simulink model "Base_Map_cs"  (R2019a)
settings: Solver=FixedStepDiscrete  StartTime=0.0  StopTime=15  FixedStep=1/300  RelTol=1e-3
PreLoadFcn:
  | mbxruntime.callbacks.PreLoadFcn(bdroot);
  | check_NUTS_defined
  | model_closed = 0;
  | assignin('base',['model_closed_' bdroot],false);
PostLoadFcn:
  | mbxruntime.callbacks.PostLoadFcn(bdroot);
InitFcn:
  | mbxruntime.callbacks.InitFcn(bdroot);
StartFcn:
  | mbxruntime.callbacks.StartFcn(bdroot);
StopFcn:
  | mbxruntime.callbacks.StopFcn(bdroot);;
  | 
model workspace: external: MAT-File .\Base_Map_S_cs_hws.mat (data not in the file)
undefined symbols (not defined in the file or in its folder): AngularVelocity, Clock_, Data, Data_SL_Info, DiscIntNeverNeededParam, Encoding, Encoding_SL_Info, Header, Height, InitImageOutputDir, LinearAcceleration, mbxruntime, Orientation, Pose, Poses, Poses_SL_Info, Position, Step, tabledata, Twist, Width
libraries: PBCSimulinkLibrary x53, robotlib x26, simulink_extras x19, PreScanSimulinkLibrary x6, dspindex x4, robotcorelib x2, sharedtransform x2, visionconversions x1, visionsinks x1
(part 3 of 8)

== system Base_Map_cs/PointCloudSensor_2 ==
  Sensor : S-Function  FunctionName=sfun_PCS  Parameters=sensorID, dataWidth, dataHeight, numChannels, dataType, timestep  SFunctionDeploymentMode=off  EnableBusSupport=off  mask(PreScan Source Block: Point Cloud Sensor){sensorID=9053, dataWidth=16, dataHeight=900, numChannels=4, dataType=0, timestep=1/20}
      mask prompts: sensorID "Sensor ID"; dataWidth "Data Width"; dataHeight "Data Height"; numChannels "Channel Count"; dataType "Data Type"; timestep "MATLAB timestep:"
      mask help: The Point Cloud Sensor provides XYZ positions relative to the sensor
      mask Help: eval('openHelp(6400)')
      mask Display: image(imread('PointCloudSensorSL.png'))
  PointCloudSensor_2 : Outport  Tag=outport/PointCloudInport  OutDataTypeStr=single  SampleTime=1/20
  wires:
  Sensor/1 -> PointCloudSensor_2/1

== system Base_Map_cs/PointCloudSensor_3 ==
  Sensor : S-Function  FunctionName=sfun_PCS  Parameters=sensorID, dataWidth, dataHeight, numChannels, dataType, timestep  SFunctionDeploymentMode=off  EnableBusSupport=off  mask(PreScan Source Block: Point Cloud Sensor){sensorID=9054, dataWidth=16, dataHeight=900, numChannels=4, dataType=0, timestep=1/20}
      mask prompts: sensorID "Sensor ID"; dataWidth "Data Width"; dataHeight "Data Height"; numChannels "Channel Count"; dataType "Data Type"; timestep "MATLAB timestep:"
      mask help: The Point Cloud Sensor provides XYZ positions relative to the sensor
      mask Help: eval('openHelp(6400)')
      mask Display: image(imread('PointCloudSensorSL.png'))
  PointCloudSensor_3 : Outport  Tag=outport/PointCloudInport  OutDataTypeStr=single  SampleTime=1/20
  wires:
  Sensor/1 -> PointCloudSensor_3/1

== system Base_Map_cs/PointCloudSensor_4 ==
  Sensor : S-Function  FunctionName=sfun_PCS  Parameters=sensorID, dataWidth, dataHeight, numChannels, dataType, timestep  SFunctionDeploymentMode=off  EnableBusSupport=off  mask(PreScan Source Block: Point Cloud Sensor){sensorID=9055, dataWidth=16, dataHeight=900, numChannels=4, dataType=0, timestep=1/20}
      mask prompts: sensorID "Sensor ID"; dataWidth "Data Width"; dataHeight "Data Height"; numChannels "Channel Count"; dataType "Data Type"; timestep "MATLAB timestep:"
      mask help: The Point Cloud Sensor provides XYZ positions relative to the sensor
      mask Help: eval('openHelp(6400)')
      mask Display: image(imread('PointCloudSensorSL.png'))
  PointCloudSensor_4 : Outport  Tag=outport/PointCloudInport  OutDataTypeStr=single  SampleTime=1/20
  wires:
  Sensor/1 -> PointCloudSensor_4/1

== system Base_Map_cs/PreScanTerminator ==
  Terminator : Terminator
  sfun_Terminator : S-Function  FunctionName=sfun_Terminator  Parameters=SampleTime  SFunctionDeploymentMode=off  EnableBusSupport=off  mask(Legacy Function){SFunctionSpec=void prescan_terminator_outputFcn(void ** work1, PRESCAN_TERMINATORDATA y1[1]), SampleTime=TimeStep, ShowSpec=on}
      mask prompts: SampleTime "Sample time (-1 for inherited):"; ShowSpec "Display function specification"
      mask help:
      | This block allows you to call the legacy functions specified by the following Legacy Code Tool definition:
      | def.SFunctionName = 'sfun_Terminator';
      | def.OutputFcnSpec = 'void prescan_terminator_outputFcn(void ** work1, PRESCAN_TERMINATORDATA y1[1])';
      | def.StartFcnSpec = 'void prescan_terminator_startFcn(void ** work1)';
      | def.TerminateFcnSpec = 'void prescan_terminator_terminateFcn(void ** work1)';
      | def.HeaderFiles = {'prescan_terminator_data.h'};
      | def.HostLibFiles = {'sensorinterfaced.lib'};
      | def.IncPaths = {'src', 'C:\prescandev\vislibrary\vis\..\pimp\include\sensors\InterfaceRTW'};
      | def.SrcPaths = {'src'};
      | def.LibPaths = {'C:\\prescandev\\vislibrary_build\lib'};
      | def.SampleTime = 'parameterized';
      | def.Options.language = 'C';
      mask Help: <p>This block was generated automatically by the Legacy Code Tool. For detailed help on this tool, call<a href="matlab:legacy_code('help')"> legacy_code('help')</a>.</p>
      mask Callback ShowSpec:
      | if strcmp(get_param(gcbh, 'ShowSpec'), 'on')
      |   set_param(gcbh, 'MaskDisplay', sprintf('fprintf(''%s'');', get_param(gcbh, 'SFunctionSpec')));
      | else
      |   set_param(gcbh, 'MaskDisplay', sprintf('fprintf(''%s'');', get_param(gcbh, 'FunctionName')));
      | end
      mask Display: fprintf('void prescan_terminator_outputFcn(void ** work1, PRESCAN_TERMINATORDATA y1[1])');
  wires:
  sfun_Terminator/1 -> Terminator/1

== system Base_Map_cs/SELF_BMW_X5_SUV_1 ==
  Sensor : S-Function  FunctionName=sfun_SelfSensor  Parameters=UniqueID, TimeStep  SFunctionDeploymentMode=off  EnableBusSupport=off  mask(PreScan Source Block: SELF){UniqueID=9040, TimeStep=1/300}
      mask prompts: UniqueID "Auto-Assigned: Unique ID"; TimeStep "Auto-Assigned: Upload Period [s]"
      mask help:
      | The SELF port shows (state) information of the actor itself. The outputs are position in the experiment's axis system and the GPS coordinates, and the object's absolute velocity and compass heading.
      |
      | For more information, please click Help.
      mask Help: eval('openHelp(462)')
      mask Display: image(imread('GPS.png'))
  SELF_BMW_X5_SUV_1 : Outport  Tag=outport/SelfPort  OutDataTypeStr=Bus: PRESCAN_SELFSENSORDATA  PortDimensions=1  SampleTime=1/300
  wires:
  Sensor/1 -> SELF_BMW_X5_SUV_1/1

== system Base_Map_cs/SELF_Citroen_C3_Hatchback_1 ==
  Sensor : S-Function  FunctionName=sfun_SelfSensor  Parameters=UniqueID, TimeStep  SFunctionDeploymentMode=off  EnableBusSupport=off  mask(PreScan Source Block: SELF){UniqueID=4877, TimeStep=1/300}
      mask prompts: UniqueID "Auto-Assigned: Unique ID"; TimeStep "Auto-Assigned: Upload Period [s]"
      mask help:
      | The SELF port shows (state) information of the actor itself. The outputs are position in the experiment's axis system and the GPS coordinates, and the object's absolute velocity and compass heading.
      |
      | For more information, please click Help.
      mask Help: eval('openHelp(462)')
      mask Display: image(imread('GPS.png'))
  SELF_Citroen_C3_Hatchback_1 : Outport  Tag=outport/SelfPort  OutDataTypeStr=Bus: PRESCAN_SELFSENSORDATA  PortDimensions=1  SampleTime=1/300
  wires:
  Sensor/1 -> SELF_Citroen_C3_Hatchback_1/1

== system Base_Map_cs/SELF_Ford_Fiesta_Hatchback_1 ==
  Sensor : S-Function  FunctionName=sfun_SelfSensor  Parameters=UniqueID, TimeStep  SFunctionDeploymentMode=off  EnableBusSupport=off  mask(PreScan Source Block: SELF){UniqueID=4876, TimeStep=1/300}
      mask prompts: UniqueID "Auto-Assigned: Unique ID"; TimeStep "Auto-Assigned: Upload Period [s]"
      mask help:
      | The SELF port shows (state) information of the actor itself. The outputs are position in the experiment's axis system and the GPS coordinates, and the object's absolute velocity and compass heading.
      |
      | For more information, please click Help.
      mask Help: eval('openHelp(462)')
      mask Display: image(imread('GPS.png'))
  SELF_Ford_Fiesta_Hatchback_1 : Outport  Tag=outport/SelfPort  OutDataTypeStr=Bus: PRESCAN_SELFSENSORDATA  PortDimensions=1  SampleTime=1/300
  wires:
  Sensor/1 -> SELF_Ford_Fiesta_Hatchback_1/1

== system Base_Map_cs/STATE_BMW_X5_SUV_1_bus ==
  STATE_BMW_X5_SUV_1_bus : Inport  Tag=inport/StatePort  OutDataTypeStr=Bus: PRESCAN_STATEACTUATORDATA  PortDimensions=1  SampleTime=1/300  BusOutputAsStruct=on
  Actuator : S-Function  FunctionName=sfun_StateActuator  Parameters=UniqueID, TimeStep  SFunctionDeploymentMode=off  EnableBusSupport=off  mask(PreScan Sink Block: State){UniqueID=9040, TimeStep=1/300}
      mask prompts: UniqueID "Auto-Assigned: Unique ID"; TimeStep "Auto-Assigned: Upload Period [s]"
      mask help:
      | The Actor State contains a vector signal of size (9x1), containing the following signals:
      |
      | -  Position    	(x,y,z)             	[m]
      | -  Velocity    	(vx,vy,vz)         	[m/s]
      | -  Angles       	(Roll, Pitch, Yaw)	[rad]
      |
      | The Actor state is defined in the global axis system.
      | The state is superponed on the Initial position defined in the GUI.
      |
      | For more information, please click Help.
      mask Help: eval('openHelp(222)')
      mask Display: image(imread('State.png'))
  wires:
  STATE_BMW_X5_SUV_1_bus/1 -> Actuator/1

== system Base_Map_cs/STATE_Citroen_C3_Hatchback_1_bus ==
  STATE_Citroen_C3_Hatchback_1_bus : Inport  Tag=inport/StatePort  OutDataTypeStr=Bus: PRESCAN_STATEACTUATORDATA  PortDimensions=1  SampleTime=1/300  BusOutputAsStruct=on
  Actuator : S-Function  FunctionName=sfun_StateActuator  Parameters=UniqueID, TimeStep  SFunctionDeploymentMode=off  EnableBusSupport=off  mask(PreScan Sink Block: State){UniqueID=4877, TimeStep=1/300}
      mask prompts: UniqueID "Auto-Assigned: Unique ID"; TimeStep "Auto-Assigned: Upload Period [s]"
      mask help:
      | The Actor State contains a vector signal of size (9x1), containing the following signals:
      |
      | -  Position    	(x,y,z)             	[m]
      | -  Velocity    	(vx,vy,vz)         	[m/s]
      | -  Angles       	(Roll, Pitch, Yaw)	[rad]
      |
      | The Actor state is defined in the global axis system.
      | The state is superponed on the Initial position defined in the GUI.
      |
      | For more information, please click Help.
      mask Help: eval('openHelp(222)')
      mask Display: image(imread('State.png'))
  wires:
  STATE_Citroen_C3_Hatchback_1_bus/1 -> Actuator/1

== system Base_Map_cs/STATE_Ford_Fiesta_Hatchback_1_bus ==
  STATE_Ford_Fiesta_Hatchback_1_bus : Inport  Tag=inport/StatePort  OutDataTypeStr=Bus: PRESCAN_STATEACTUATORDATA  PortDimensions=1  SampleTime=1/300  BusOutputAsStruct=on
  Actuator : S-Function  FunctionName=sfun_StateActuator  Parameters=UniqueID, TimeStep  SFunctionDeploymentMode=off  EnableBusSupport=off  mask(PreScan Sink Block: State){UniqueID=4876, TimeStep=1/300}
      mask prompts: UniqueID "Auto-Assigned: Unique ID"; TimeStep "Auto-Assigned: Upload Period [s]"
      mask help:
      | The Actor State contains a vector signal of size (9x1), containing the following signals:
      |
      | -  Position    	(x,y,z)             	[m]
      | -  Velocity    	(vx,vy,vz)         	[m/s]
      | -  Angles       	(Roll, Pitch, Yaw)	[rad]
      |
      | The Actor state is defined in the global axis system.
      | The state is superponed on the Initial position defined in the GUI.
      |
      | For more information, please click Help.
      mask Help: eval('openHelp(222)')
      mask Display: image(imread('State.png'))
  wires:
  STATE_Ford_Fiesta_Hatchback_1_bus/1 -> Actuator/1

== system Base_Map_cs/Synchronizer ==
  Bus Selector1 : BusSelector  OutputSignals=FederateStopped
  Stop Simulation : Stop
  sfun_Synchronizer : S-Function  FunctionName=sfun_Synchronizer  Parameters=SampleTime  SFunctionDeploymentMode=off  EnableBusSupport=off  mask(Legacy Function){SFunctionSpec=void prescan_synchronizer_outputFcn(void ** work1, PRESCAN_SYNCHRONIZEDATA y1[1]), SampleTime=TimeStep, ShowSpec=on}
      mask prompts: SampleTime "Sample time (-1 for inherited):"; ShowSpec "Display function specification"
      mask help:
      | This block allows you to call the legacy functions specified by the following Legacy Code Tool definition:
      | def.SFunctionName = 'sfun_Synchronizer';
      | def.OutputFcnSpec = 'void prescan_synchronizer_outputFcn(void ** work1, PRESCAN_SYNCHRONIZEDATA y1[1])';
      | def.StartFcnSpec = 'void prescan_synchronizer_startFcn(void ** work1)';
      | def.TerminateFcnSpec = 'void prescan_synchronizer_terminateFcn(void ** work1)';
      | def.HeaderFiles = {'prescan_synchronizer_data.h'};
      | def.HostLibFiles = {'sensorinterfaced.lib'};
      | def.IncPaths = {'src', 'C:\prescandev\vislibrary\vis\..\pimp\include\sensors\InterfaceRTW'};
      | def.SrcPaths = {'src'};
      | def.LibPaths = {'C:\\prescandev\\vislibrary_build\lib'};
      | def.SampleTime = 'parameterized';
      | def.Options.language = 'C';
      mask Help: <p>This block was generated automatically by the Legacy Code Tool. For detailed help on this tool, call<a href="matlab:legacy_code('help')"> legacy_code('help')</a>.</p>
      mask Callback ShowSpec:
      | if strcmp(get_param(gcbh, 'ShowSpec'), 'on')
      |   set_param(gcbh, 'MaskDisplay', sprintf('fprintf(''%s'');', get_param(gcbh, 'SFunctionSpec')));
      | else
      |   set_param(gcbh, 'MaskDisplay', sprintf('fprintf(''%s'');', get_param(gcbh, 'FunctionName')));
      | end
      mask Display: fprintf('void prescan_synchronizer_outputFcn(void ** work1, PRESCAN_SYNCHRONIZEDATA y1[1])');
  wires:
  Bus Selector1/1 -> Stop Simulation/1  "<FederateStopped>"
  sfun_Synchronizer/1 -> Bus Selector1/1

== system Base_Map_cs/TrafficLightRoadSideNL_1 ==
  note: Light SPD Resources
      |
      |  0: CIE_A_standard_incandescent_illuminant.txt
      |  1: CIE_A_standard_incandescent_illuminant.txt_x_R255_G191_B000.txt
      |  2: CIE_A_standard_incandescent_illuminant.txt_x_R583_G047_B000.txt
      |  3: CIE_F12_standard_fluorescent_illuminant.txt
      |  4: Illuminant_D65.txt
      |  5: Light_SPD_H1_12_8V_Filament.txt
      |  6: Light_SPD_H1_13_2V_Filament.txt
      |  7: Light_SPD_H11_12V_Filament.txt
      |  8: Light_SPD_H7_12_8V_Filament.txt
      |  9: Light_SPD_H7_13_2V_Filament.txt
      | 10: Light_SPD_H8_13_2V_Filament.txt
      | 11: Light_SPD_Halogen.txt
      | 12: Light_SPD_High_Power_LED.txt
      | 13: Light_SPD_HPS_High_Pressure_Sodium.txt
      | 14: Light_SPD_incandescent_traffic_signal_amber.txt
      | 15: Light_SPD_incandescent_traffic_signal_green.txt
      | 16: Light_SPD_incandescent_traffic_signal_red.txt
      | 17: Light_SPD_LED_D1S_HID.txt
      | 18: Light_SPD_LED_traffic_signal_amber.txt
      | 19: Light_SPD_LED_traffic_signal_green.txt
      | 20: Light_SPD_LED_traffic_signal_red.txt
      | 21: Light_SPD_LPS_Low_Pressure_Sodium.txt
      | 22: Light_SPD_Mercury.txt
      | 23: Light_SPD_Reddish_Neon_Sign.txt
      | 24: Noma_Twister_Blue_13W_120V.txt
      | 25: Philips_Blue_Golite_P1_Apollo_1750Lux.txt
      | 26: SPD_flat_1.0.txt
  note: Light SPD Resources
  Ground_1 : Ground
  Ground_2 : Ground
  Ground_3 : Ground
  TrafficLightRoadSideNL_1_Casing.LightGreen_Control_Mux : Subsystem  Tag=mux/plugin/LightSignals
  TrafficLightRoadSideNL_1_Casing.LightGreen_Power : Constant  Tag=TrafficLightRoadSideNL_1_Casing.LightGreen_Power  Value=0
  TrafficLightRoadSideNL_1_Casing.LightGreen_SPDIndex : Constant  Tag=TrafficLightRoadSideNL_1_Casing.LightGreen_SPDIndex  Value=15
  TrafficLightRoadSideNL_1_Casing.LightOrange_Control_Mux : Subsystem  Tag=mux/plugin/LightSignals
  TrafficLightRoadSideNL_1_Casing.LightOrange_Power : Constant  Tag=TrafficLightRoadSideNL_1_Casing.LightOrange_Power  Value=0
  TrafficLightRoadSideNL_1_Casing.LightOrange_SPDIndex : Constant  Tag=TrafficLightRoadSideNL_1_Casing.LightOrange_SPDIndex  Value=14
  TrafficLightRoadSideNL_1_Casing.LightRed_Control_Mux : Subsystem  Tag=mux/plugin/LightSignals
  TrafficLightRoadSideNL_1_Casing.LightRed_Power : Constant  Tag=TrafficLightRoadSideNL_1_Casing.LightRed_Power  Value=0
  TrafficLightRoadSideNL_1_Casing.LightRed_SPDIndex : Constant  Tag=TrafficLightRoadSideNL_1_Casing.LightRed_SPDIndex  Value=16
  VISUCasingLights_Mux : Subsystem  Tag=mux/VisuCasingLights  mask(PreScan User Interface: VisuTrafficLight){}
      mask help:
      | The VisuTrafficLight block provides a way to animate traffic lights: switch on and off individual lights.
      |
      | For more information, please click Help.
      mask Help: eval('openHelp(731)')
  VISUCasingLights_TrafficLightRoadSideNL_1 : Outport  Tag=outport/VisuCasingLights  SampleTime=1/300
  TrafficLightRoadSideNL_1_Casing.LightRed_Control : Outport  Tag=outport/plugin/sfun_PBCLight  Port=2  OutDataTypeStr=Bus: PRESCAN_PBCLIGHT_DATA  PortDimensions=1  SampleTime=0.05
  TrafficLightRoadSideNL_1_Casing.LightOrange_Control : Outport  Tag=outport/plugin/sfun_PBCLight  Port=3  OutDataTypeStr=Bus: PRESCAN_PBCLIGHT_DATA  PortDimensions=1  SampleTime=0.05
  TrafficLightRoadSideNL_1_Casing.LightGreen_Control : Outport  Tag=outport/plugin/sfun_PBCLight  Port=4  OutDataTypeStr=Bus: PRESCAN_PBCLIGHT_DATA  PortDimensions=1  SampleTime=0.05
  wires:
  VISUCasingLights_Mux/1(VISUCasingLights_TrafficLightRoadSideNL_1) -> VISUCasingLights_TrafficLightRoadSideNL_1/1
  TrafficLightRoadSideNL_1_Casing.LightRed_Control_Mux/1(Bus) -> TrafficLightRoadSideNL_1_Casing.LightRed_Control/1
  TrafficLightRoadSideNL_1_Casing.LightRed_SPDIndex/1 -> TrafficLightRoadSideNL_1_Casing.LightRed_Control_Mux/1(SPDIndex [-])
  TrafficLightRoadSideNL_1_Casing.LightRed_Power/1 -> TrafficLightRoadSideNL_1_Casing.LightRed_Control_Mux/2(Power [W])
  TrafficLightRoadSideNL_1_Casing.LightOrange_Control_Mux/1(Bus) -> TrafficLightRoadSideNL_1_Casing.LightOrange_Control/1
  TrafficLightRoadSideNL_1_Casing.LightOrange_SPDIndex/1 -> TrafficLightRoadSideNL_1_Casing.LightOrange_Control_Mux/1(SPDIndex [-])
  TrafficLightRoadSideNL_1_Casing.LightOrange_Power/1 -> TrafficLightRoadSideNL_1_Casing.LightOrange_Control_Mux/2(Power [W])
  TrafficLightRoadSideNL_1_Casing.LightGreen_Control_Mux/1(Bus) -> TrafficLightRoadSideNL_1_Casing.LightGreen_Control/1
  TrafficLightRoadSideNL_1_Casing.LightGreen_SPDIndex/1 -> TrafficLightRoadSideNL_1_Casing.LightGreen_Control_Mux/1(SPDIndex [-])
  TrafficLightRoadSideNL_1_Casing.LightGreen_Power/1 -> TrafficLightRoadSideNL_1_Casing.LightGreen_Control_Mux/2(Power [W])
  Ground_1/1 -> VISUCasingLights_Mux/1(Green [-])
  Ground_2/1 -> VISUCasingLights_Mux/2(Orange [-])
  Ground_3/1 -> VISUCasingLights_Mux/3(Red [-])

== system Base_Map_cs/TrafficLightRoadSideNL_1_Casing.LightGreen_Control ==
  TrafficLightRoadSideNL_1_Casing.LightGreen_Control : Inport  Tag=inport/plugin/sfun_PBCLight  OutDataTypeStr=Bus: PRESCAN_PBCLIGHT_DATA  PortDimensions=1  SampleTime=0.05  BusOutputAsStruct=on
  Actuator : S-Function  LoadFcn=addpath 'C:/Program Files/Simcenter Prescan/Prescan_2019.1/Plugins/PBCameraPlugin/matlab';addpath 'C:/Program Files/Simcenter Prescan/Prescan_2019.1/Plugins/PBCameraPlugin/bin';load('PreScanPBCLightData.mat');  FunctionName=sfun_PBCLight  Parameters=lightID, timestepMask  SFunctionDeploymentMode=off  EnableBusSupport=off  mask(Physics Based Camera plugin block){lightID=2, timestepMask=0.05}
      mask prompts: lightID "Light ID:"; timestepMask "MATLAB timestep:"
      mask help: Light Control I/O
      mask Help: eval('openHelp(6500)')
      mask Display: image(imread('ico_PBCControl.png'))
  wires:
  TrafficLightRoadSideNL_1_Casing.LightGreen_Control/1 -> Actuator/1

== system Base_Map_cs/TrafficLightRoadSideNL_1_Casing.LightOrange_Control ==
  TrafficLightRoadSideNL_1_Casing.LightOrange_Control : Inport  Tag=inport/plugin/sfun_PBCLight  OutDataTypeStr=Bus: PRESCAN_PBCLIGHT_DATA  PortDimensions=1  SampleTime=0.05  BusOutputAsStruct=on
  Actuator : S-Function  LoadFcn=addpath 'C:/Program Files/Simcenter Prescan/Prescan_2019.1/Plugins/PBCameraPlugin/matlab';addpath 'C:/Program Files/Simcenter Prescan/Prescan_2019.1/Plugins/PBCameraPlugin/bin';load('PreScanPBCLightData.mat');  FunctionName=sfun_PBCLight  Parameters=lightID, timestepMask  SFunctionDeploymentMode=off  EnableBusSupport=off  mask(Physics Based Camera plugin block){lightID=1, timestepMask=0.05}
      mask prompts: lightID "Light ID:"; timestepMask "MATLAB timestep:"
      mask help: Light Control I/O
      mask Help: eval('openHelp(6500)')
      mask Display: image(imread('ico_PBCControl.png'))
  wires:
  TrafficLightRoadSideNL_1_Casing.LightOrange_Control/1 -> Actuator/1

== system Base_Map_cs/TrafficLightRoadSideNL_1_Casing.LightRed_Control ==
  TrafficLightRoadSideNL_1_Casing.LightRed_Control : Inport  Tag=inport/plugin/sfun_PBCLight  OutDataTypeStr=Bus: PRESCAN_PBCLIGHT_DATA  PortDimensions=1  SampleTime=0.05  BusOutputAsStruct=on
  Actuator : S-Function  LoadFcn=addpath 'C:/Program Files/Simcenter Prescan/Prescan_2019.1/Plugins/PBCameraPlugin/matlab';addpath 'C:/Program Files/Simcenter Prescan/Prescan_2019.1/Plugins/PBCameraPlugin/bin';load('PreScanPBCLightData.mat');  FunctionName=sfun_PBCLight  Parameters=lightID, timestepMask  SFunctionDeploymentMode=off  EnableBusSupport=off  mask(Physics Based Camera plugin block){lightID=0, timestepMask=0.05}
      mask prompts: lightID "Light ID:"; timestepMask "MATLAB timestep:"
      mask help: Light Control I/O
      mask Help: eval('openHelp(6500)')
      mask Display: image(imread('ico_PBCControl.png'))
  wires:
  TrafficLightRoadSideNL_1_Casing.LightRed_Control/1 -> Actuator/1

== system Base_Map_cs/TrafficLightRoadSideNL_2 ==
  note: Light SPD Resources
      |
      |  0: CIE_A_standard_incandescent_illuminant.txt
      |  1: CIE_A_standard_incandescent_illuminant.txt_x_R255_G191_B000.txt
      |  2: CIE_A_standard_incandescent_illuminant.txt_x_R583_G047_B000.txt
      |  3: CIE_F12_standard_fluorescent_illuminant.txt
      |  4: Illuminant_D65.txt
      |  5: Light_SPD_H1_12_8V_Filament.txt
      |  6: Light_SPD_H1_13_2V_Filament.txt
      |  7: Light_SPD_H11_12V_Filament.txt
      |  8: Light_SPD_H7_12_8V_Filament.txt
      |  9: Light_SPD_H7_13_2V_Filament.txt
      | 10: Light_SPD_H8_13_2V_Filament.txt
      | 11: Light_SPD_Halogen.txt
      | 12: Light_SPD_High_Power_LED.txt
      | 13: Light_SPD_HPS_High_Pressure_Sodium.txt
      | 14: Light_SPD_incandescent_traffic_signal_amber.txt
      | 15: Light_SPD_incandescent_traffic_signal_green.txt
      | 16: Light_SPD_incandescent_traffic_signal_red.txt
      | 17: Light_SPD_LED_D1S_HID.txt
      | 18: Light_SPD_LED_traffic_signal_amber.txt
      | 19: Light_SPD_LED_traffic_signal_green.txt
      | 20: Light_SPD_LED_traffic_signal_red.txt
      | 21: Light_SPD_LPS_Low_Pressure_Sodium.txt
      | 22: Light_SPD_Mercury.txt
      | 23: Light_SPD_Reddish_Neon_Sign.txt
      | 24: Noma_Twister_Blue_13W_120V.txt
      | 25: Philips_Blue_Golite_P1_Apollo_1750Lux.txt
      | 26: SPD_flat_1.0.txt
  note: Light SPD Resources
  Ground_1 : Ground
  Ground_2 : Ground
  Ground_3 : Ground
  TrafficLightRoadSideNL_2_Casing.LightGreen_Control_Mux : Subsystem  Tag=mux/plugin/LightSignals
  TrafficLightRoadSideNL_2_Casing.LightGreen_Power : Constant  Tag=TrafficLightRoadSideNL_2_Casing.LightGreen_Power  Value=0
  TrafficLightRoadSideNL_2_Casing.LightGreen_SPDIndex : Constant  Tag=TrafficLightRoadSideNL_2_Casing.LightGreen_SPDIndex  Value=15
  TrafficLightRoadSideNL_2_Casing.LightOrange_Control_Mux : Subsystem  Tag=mux/plugin/LightSignals
  TrafficLightRoadSideNL_2_Casing.LightOrange_Power : Constant  Tag=TrafficLightRoadSideNL_2_Casing.LightOrange_Power  Value=0
  TrafficLightRoadSideNL_2_Casing.LightOrange_SPDIndex : Constant  Tag=TrafficLightRoadSideNL_2_Casing.LightOrange_SPDIndex  Value=14
  TrafficLightRoadSideNL_2_Casing.LightRed_Control_Mux : Subsystem  Tag=mux/plugin/LightSignals
  TrafficLightRoadSideNL_2_Casing.LightRed_Power : Constant  Tag=TrafficLightRoadSideNL_2_Casing.LightRed_Power  Value=0
  TrafficLightRoadSideNL_2_Casing.LightRed_SPDIndex : Constant  Tag=TrafficLightRoadSideNL_2_Casing.LightRed_SPDIndex  Value=16
  VISUCasingLights_Mux : Subsystem  Tag=mux/VisuCasingLights  mask(PreScan User Interface: VisuTrafficLight){}
      mask help:
      | The VisuTrafficLight block provides a way to animate traffic lights: switch on and off individual lights.
      |
      | For more information, please click Help.
      mask Help: eval('openHelp(731)')
  VISUCasingLights_TrafficLightRoadSideNL_2 : Outport  Tag=outport/VisuCasingLights  SampleTime=1/300
  TrafficLightRoadSideNL_2_Casing.LightRed_Control : Outport  Tag=outport/plugin/sfun_PBCLight  Port=2  OutDataTypeStr=Bus: PRESCAN_PBCLIGHT_DATA  PortDimensions=1  SampleTime=0.05
  TrafficLightRoadSideNL_2_Casing.LightOrange_Control : Outport  Tag=outport/plugin/sfun_PBCLight  Port=3  OutDataTypeStr=Bus: PRESCAN_PBCLIGHT_DATA  PortDimensions=1  SampleTime=0.05
  TrafficLightRoadSideNL_2_Casing.LightGreen_Control : Outport  Tag=outport/plugin/sfun_PBCLight  Port=4  OutDataTypeStr=Bus: PRESCAN_PBCLIGHT_DATA  PortDimensions=1  SampleTime=0.05
  wires:
  VISUCasingLights_Mux/1(VISUCasingLights_TrafficLightRoadSideNL_2) -> VISUCasingLights_TrafficLightRoadSideNL_2/1
  TrafficLightRoadSideNL_2_Casing.LightRed_Control_Mux/1(Bus) -> TrafficLightRoadSideNL_2_Casing.LightRed_Control/1
  TrafficLightRoadSideNL_2_Casing.LightRed_SPDIndex/1 -> TrafficLightRoadSideNL_2_Casing.LightRed_Control_Mux/1(SPDIndex [-])
  TrafficLightRoadSideNL_2_Casing.LightRed_Power/1 -> TrafficLightRoadSideNL_2_Casing.LightRed_Control_Mux/2(Power [W])
  TrafficLightRoadSideNL_2_Casing.LightOrange_Control_Mux/1(Bus) -> TrafficLightRoadSideNL_2_Casing.LightOrange_Control/1
  TrafficLightRoadSideNL_2_Casing.LightOrange_SPDIndex/1 -> TrafficLightRoadSideNL_2_Casing.LightOrange_Control_Mux/1(SPDIndex [-])
  TrafficLightRoadSideNL_2_Casing.LightOrange_Power/1 -> TrafficLightRoadSideNL_2_Casing.LightOrange_Control_Mux/2(Power [W])
  TrafficLightRoadSideNL_2_Casing.LightGreen_Control_Mux/1(Bus) -> TrafficLightRoadSideNL_2_Casing.LightGreen_Control/1
  TrafficLightRoadSideNL_2_Casing.LightGreen_SPDIndex/1 -> TrafficLightRoadSideNL_2_Casing.LightGreen_Control_Mux/1(SPDIndex [-])
  TrafficLightRoadSideNL_2_Casing.LightGreen_Power/1 -> TrafficLightRoadSideNL_2_Casing.LightGreen_Control_Mux/2(Power [W])
  Ground_1/1 -> VISUCasingLights_Mux/1(Green [-])
  Ground_2/1 -> VISUCasingLights_Mux/2(Orange [-])
  Ground_3/1 -> VISUCasingLights_Mux/3(Red [-])

== system Base_Map_cs/TrafficLightRoadSideNL_2_Casing.LightGreen_Control ==
  TrafficLightRoadSideNL_2_Casing.LightGreen_Control : Inport  Tag=inport/plugin/sfun_PBCLight  OutDataTypeStr=Bus: PRESCAN_PBCLIGHT_DATA  PortDimensions=1  SampleTime=0.05  BusOutputAsStruct=on
  Actuator : S-Function  LoadFcn=addpath 'C:/Program Files/Simcenter Prescan/Prescan_2019.1/Plugins/PBCameraPlugin/matlab';addpath 'C:/Program Files/Simcenter Prescan/Prescan_2019.1/Plugins/PBCameraPlugin/bin';load('PreScanPBCLightData.mat');  FunctionName=sfun_PBCLight  Parameters=lightID, timestepMask  SFunctionDeploymentMode=off  EnableBusSupport=off  mask(Physics Based Camera plugin block){lightID=5, timestepMask=0.05}
      mask prompts: lightID "Light ID:"; timestepMask "MATLAB timestep:"
      mask help: Light Control I/O
      mask Help: eval('openHelp(6500)')
      mask Display: image(imread('ico_PBCControl.png'))
  wires:
  TrafficLightRoadSideNL_2_Casing.LightGreen_Control/1 -> Actuator/1

== system Base_Map_cs/TrafficLightRoadSideNL_2_Casing.LightOrange_Control ==
  TrafficLightRoadSideNL_2_Casing.LightOrange_Control : Inport  Tag=inport/plugin/sfun_PBCLight  OutDataTypeStr=Bus: PRESCAN_PBCLIGHT_DATA  PortDimensions=1  SampleTime=0.05  BusOutputAsStruct=on
  Actuator : S-Function  LoadFcn=addpath 'C:/Program Files/Simcenter Prescan/Prescan_2019.1/Plugins/PBCameraPlugin/matlab';addpath 'C:/Program Files/Simcenter Prescan/Prescan_2019.1/Plugins/PBCameraPlugin/bin';load('PreScanPBCLightData.mat');  FunctionName=sfun_PBCLight  Parameters=lightID, timestepMask  SFunctionDeploymentMode=off  EnableBusSupport=off  mask(Physics Based Camera plugin block){lightID=4, timestepMask=0.05}
      mask prompts: lightID "Light ID:"; timestepMask "MATLAB timestep:"
      mask help: Light Control I/O
      mask Help: eval('openHelp(6500)')
      mask Display: image(imread('ico_PBCControl.png'))
  wires:
  TrafficLightRoadSideNL_2_Casing.LightOrange_Control/1 -> Actuator/1

== system Base_Map_cs/TrafficLightRoadSideNL_2_Casing.LightRed_Control ==
  TrafficLightRoadSideNL_2_Casing.LightRed_Control : Inport  Tag=inport/plugin/sfun_PBCLight  OutDataTypeStr=Bus: PRESCAN_PBCLIGHT_DATA  PortDimensions=1  SampleTime=0.05  BusOutputAsStruct=on
  Actuator : S-Function  LoadFcn=addpath 'C:/Program Files/Simcenter Prescan/Prescan_2019.1/Plugins/PBCameraPlugin/matlab';addpath 'C:/Program Files/Simcenter Prescan/Prescan_2019.1/Plugins/PBCameraPlugin/bin';load('PreScanPBCLightData.mat');  FunctionName=sfun_PBCLight  Parameters=lightID, timestepMask  SFunctionDeploymentMode=off  EnableBusSupport=off  mask(Physics Based Camera plugin block){lightID=3, timestepMask=0.05}
      mask prompts: lightID "Light ID:"; timestepMask "MATLAB timestep:"
      mask help: Light Control I/O
      mask Help: eval('openHelp(6500)')
      mask Display: image(imread('ico_PBCControl.png'))
  wires:
  TrafficLightRoadSideNL_2_Casing.LightRed_Control/1 -> Actuator/1

== system Base_Map_cs/TrafficLightRoadSideNL_3 ==
  note: Light SPD Resources
      |
      |  0: CIE_A_standard_incandescent_illuminant.txt
      |  1: CIE_A_standard_incandescent_illuminant.txt_x_R255_G191_B000.txt
      |  2: CIE_A_standard_incandescent_illuminant.txt_x_R583_G047_B000.txt
      |  3: CIE_F12_standard_fluorescent_illuminant.txt
      |  4: Illuminant_D65.txt
      |  5: Light_SPD_H1_12_8V_Filament.txt
      |  6: Light_SPD_H1_13_2V_Filament.txt
      |  7: Light_SPD_H11_12V_Filament.txt
      |  8: Light_SPD_H7_12_8V_Filament.txt
      |  9: Light_SPD_H7_13_2V_Filament.txt
      | 10: Light_SPD_H8_13_2V_Filament.txt
      | 11: Light_SPD_Halogen.txt
      | 12: Light_SPD_High_Power_LED.txt
      | 13: Light_SPD_HPS_High_Pressure_Sodium.txt
      | 14: Light_SPD_incandescent_traffic_signal_amber.txt
      | 15: Light_SPD_incandescent_traffic_signal_green.txt
      | 16: Light_SPD_incandescent_traffic_signal_red.txt
      | 17: Light_SPD_LED_D1S_HID.txt
      | 18: Light_SPD_LED_traffic_signal_amber.txt
      | 19: Light_SPD_LED_traffic_signal_green.txt
      | 20: Light_SPD_LED_traffic_signal_red.txt
      | 21: Light_SPD_LPS_Low_Pressure_Sodium.txt
      | 22: Light_SPD_Mercury.txt
      | 23: Light_SPD_Reddish_Neon_Sign.txt
      | 24: Noma_Twister_Blue_13W_120V.txt
      | 25: Philips_Blue_Golite_P1_Apollo_1750Lux.txt
      | 26: SPD_flat_1.0.txt
  note: Light SPD Resources
  Ground_1 : Ground
  Ground_2 : Ground
  Ground_3 : Ground
  TrafficLightRoadSideNL_3_Casing.LightGreen_Control_Mux : Subsystem  Tag=mux/plugin/LightSignals
  TrafficLightRoadSideNL_3_Casing.LightGreen_Power : Constant  Tag=TrafficLightRoadSideNL_3_Casing.LightGreen_Power  Value=0
  TrafficLightRoadSideNL_3_Casing.LightGreen_SPDIndex : Constant  Tag=TrafficLightRoadSideNL_3_Casing.LightGreen_SPDIndex  Value=15
  TrafficLightRoadSideNL_3_Casing.LightOrange_Control_Mux : Subsystem  Tag=mux/plugin/LightSignals
  TrafficLightRoadSideNL_3_Casing.LightOrange_Power : Constant  Tag=TrafficLightRoadSideNL_3_Casing.LightOrange_Power  Value=0
  TrafficLightRoadSideNL_3_Casing.LightOrange_SPDIndex : Constant  Tag=TrafficLightRoadSideNL_3_Casing.LightOrange_SPDIndex  Value=14
  TrafficLightRoadSideNL_3_Casing.LightRed_Control_Mux : Subsystem  Tag=mux/plugin/LightSignals
  TrafficLightRoadSideNL_3_Casing.LightRed_Power : Constant  Tag=TrafficLightRoadSideNL_3_Casing.LightRed_Power  Value=0
  TrafficLightRoadSideNL_3_Casing.LightRed_SPDIndex : Constant  Tag=TrafficLightRoadSideNL_3_Casing.LightRed_SPDIndex  Value=16
  VISUCasingLights_Mux : Subsystem  Tag=mux/VisuCasingLights  mask(PreScan User Interface: VisuTrafficLight){}
      mask help:
      | The VisuTrafficLight block provides a way to animate traffic lights: switch on and off individual lights.
      |
      | For more information, please click Help.
      mask Help: eval('openHelp(731)')
  VISUCasingLights_TrafficLightRoadSideNL_3 : Outport  Tag=outport/VisuCasingLights  SampleTime=1/300
  TrafficLightRoadSideNL_3_Casing.LightRed_Control : Outport  Tag=outport/plugin/sfun_PBCLight  Port=2  OutDataTypeStr=Bus: PRESCAN_PBCLIGHT_DATA  PortDimensions=1  SampleTime=0.05
  TrafficLightRoadSideNL_3_Casing.LightOrange_Control : Outport  Tag=outport/plugin/sfun_PBCLight  Port=3  OutDataTypeStr=Bus: PRESCAN_PBCLIGHT_DATA  PortDimensions=1  SampleTime=0.05
  TrafficLightRoadSideNL_3_Casing.LightGreen_Control : Outport  Tag=outport/plugin/sfun_PBCLight  Port=4  OutDataTypeStr=Bus: PRESCAN_PBCLIGHT_DATA  PortDimensions=1  SampleTime=0.05
  wires:
  VISUCasingLights_Mux/1(VISUCasingLights_TrafficLightRoadSideNL_3) -> VISUCasingLights_TrafficLightRoadSideNL_3/1
  TrafficLightRoadSideNL_3_Casing.LightRed_Control_Mux/1(Bus) -> TrafficLightRoadSideNL_3_Casing.LightRed_Control/1
  TrafficLightRoadSideNL_3_Casing.LightRed_SPDIndex/1 -> TrafficLightRoadSideNL_3_Casing.LightRed_Control_Mux/1(SPDIndex [-])
  TrafficLightRoadSideNL_3_Casing.LightRed_Power/1 -> TrafficLightRoadSideNL_3_Casing.LightRed_Control_Mux/2(Power [W])
  TrafficLightRoadSideNL_3_Casing.LightOrange_Control_Mux/1(Bus) -> TrafficLightRoadSideNL_3_Casing.LightOrange_Control/1
  TrafficLightRoadSideNL_3_Casing.LightOrange_SPDIndex/1 -> TrafficLightRoadSideNL_3_Casing.LightOrange_Control_Mux/1(SPDIndex [-])
  TrafficLightRoadSideNL_3_Casing.LightOrange_Power/1 -> TrafficLightRoadSideNL_3_Casing.LightOrange_Control_Mux/2(Power [W])
  TrafficLightRoadSideNL_3_Casing.LightGreen_Control_Mux/1(Bus) -> TrafficLightRoadSideNL_3_Casing.LightGreen_Control/1
  TrafficLightRoadSideNL_3_Casing.LightGreen_SPDIndex/1 -> TrafficLightRoadSideNL_3_Casing.LightGreen_Control_Mux/1(SPDIndex [-])
  TrafficLightRoadSideNL_3_Casing.LightGreen_Power/1 -> TrafficLightRoadSideNL_3_Casing.LightGreen_Control_Mux/2(Power [W])
  Ground_1/1 -> VISUCasingLights_Mux/1(Green [-])
  Ground_2/1 -> VISUCasingLights_Mux/2(Orange [-])
  Ground_3/1 -> VISUCasingLights_Mux/3(Red [-])

== system Base_Map_cs/TrafficLightRoadSideNL_3_Casing.LightGreen_Control ==
  TrafficLightRoadSideNL_3_Casing.LightGreen_Control : Inport  Tag=inport/plugin/sfun_PBCLight  OutDataTypeStr=Bus: PRESCAN_PBCLIGHT_DATA  PortDimensions=1  SampleTime=0.05  BusOutputAsStruct=on
  Actuator : S-Function  LoadFcn=addpath 'C:/Program Files/Simcenter Prescan/Prescan_2019.1/Plugins/PBCameraPlugin/matlab';addpath 'C:/Program Files/Simcenter Prescan/Prescan_2019.1/Plugins/PBCameraPlugin/bin';load('PreScanPBCLightData.mat');  FunctionName=sfun_PBCLight  Parameters=lightID, timestepMask  SFunctionDeploymentMode=off  EnableBusSupport=off  mask(Physics Based Camera plugin block){lightID=8, timestepMask=0.05}
      mask prompts: lightID "Light ID:"; timestepMask "MATLAB timestep:"
      mask help: Light Control I/O
      mask Help: eval('openHelp(6500)')
      mask Display: image(imread('ico_PBCControl.png'))
  wires:
  TrafficLightRoadSideNL_3_Casing.LightGreen_Control/1 -> Actuator/1

== system Base_Map_cs/TrafficLightRoadSideNL_3_Casing.LightOrange_Control ==
  TrafficLightRoadSideNL_3_Casing.LightOrange_Control : Inport  Tag=inport/plugin/sfun_PBCLight  OutDataTypeStr=Bus: PRESCAN_PBCLIGHT_DATA  PortDimensions=1  SampleTime=0.05  BusOutputAsStruct=on
  Actuator : S-Function  LoadFcn=addpath 'C:/Program Files/Simcenter Prescan/Prescan_2019.1/Plugins/PBCameraPlugin/matlab';addpath 'C:/Program Files/Simcenter Prescan/Prescan_2019.1/Plugins/PBCameraPlugin/bin';load('PreScanPBCLightData.mat');  FunctionName=sfun_PBCLight  Parameters=lightID, timestepMask  SFunctionDeploymentMode=off  EnableBusSupport=off  mask(Physics Based Camera plugin block){lightID=7, timestepMask=0.05}
      mask prompts: lightID "Light ID:"; timestepMask "MATLAB timestep:"
      mask help: Light Control I/O
      mask Help: eval('openHelp(6500)')
      mask Display: image(imread('ico_PBCControl.png'))
  wires:
  TrafficLightRoadSideNL_3_Casing.LightOrange_Control/1 -> Actuator/1

== system Base_Map_cs/TrafficLightRoadSideNL_3_Casing.LightRed_Control ==
  TrafficLightRoadSideNL_3_Casing.LightRed_Control : Inport  Tag=inport/plugin/sfun_PBCLight  OutDataTypeStr=Bus: PRESCAN_PBCLIGHT_DATA  PortDimensions=1  SampleTime=0.05  BusOutputAsStruct=on
  Actuator : S-Function  LoadFcn=addpath 'C:/Program Files/Simcenter Prescan/Prescan_2019.1/Plugins/PBCameraPlugin/matlab';addpath 'C:/Program Files/Simcenter Prescan/Prescan_2019.1/Plugins/PBCameraPlugin/bin';load('PreScanPBCLightData.mat');  FunctionName=sfun_PBCLight  Parameters=lightID, timestepMask  SFunctionDeploymentMode=off  EnableBusSupport=off  mask(Physics Based Camera plugin block){lightID=6, timestepMask=0.05}
      mask prompts: lightID "Light ID:"; timestepMask "MATLAB timestep:"
      mask help: Light Control I/O
      mask Help: eval('openHelp(6500)')
      mask Display: image(imread('ico_PBCControl.png'))
  wires:
  TrafficLightRoadSideNL_3_Casing.LightRed_Control/1 -> Actuator/1

== system Base_Map_cs/TrafficLightRoadSideNL_4 ==
  note: Light SPD Resources
      |
      |  0: CIE_A_standard_incandescent_illuminant.txt
      |  1: CIE_A_standard_incandescent_illuminant.txt_x_R255_G191_B000.txt
      |  2: CIE_A_standard_incandescent_illuminant.txt_x_R583_G047_B000.txt
      |  3: CIE_F12_standard_fluorescent_illuminant.txt
      |  4: Illuminant_D65.txt
      |  5: Light_SPD_H1_12_8V_Filament.txt
      |  6: Light_SPD_H1_13_2V_Filament.txt
      |  7: Light_SPD_H11_12V_Filament.txt
      |  8: Light_SPD_H7_12_8V_Filament.txt
      |  9: Light_SPD_H7_13_2V_Filament.txt
      | 10: Light_SPD_H8_13_2V_Filament.txt
      | 11: Light_SPD_Halogen.txt
      | 12: Light_SPD_High_Power_LED.txt
      | 13: Light_SPD_HPS_High_Pressure_Sodium.txt
      | 14: Light_SPD_incandescent_traffic_signal_amber.txt
      | 15: Light_SPD_incandescent_traffic_signal_green.txt
      | 16: Light_SPD_incandescent_traffic_signal_red.txt
      | 17: Light_SPD_LED_D1S_HID.txt
      | 18: Light_SPD_LED_traffic_signal_amber.txt
      | 19: Light_SPD_LED_traffic_signal_green.txt
      | 20: Light_SPD_LED_traffic_signal_red.txt
      | 21: Light_SPD_LPS_Low_Pressure_Sodium.txt
      | 22: Light_SPD_Mercury.txt
      | 23: Light_SPD_Reddish_Neon_Sign.txt
      | 24: Noma_Twister_Blue_13W_120V.txt
      | 25: Philips_Blue_Golite_P1_Apollo_1750Lux.txt
      | 26: SPD_flat_1.0.txt
  note: Light SPD Resources
  Ground_1 : Ground
  Ground_2 : Ground
  Ground_3 : Ground
  TrafficLightRoadSideNL_4_Casing.LightGreen_Control_Mux : Subsystem  Tag=mux/plugin/LightSignals
  TrafficLightRoadSideNL_4_Casing.LightGreen_Power : Constant  Tag=TrafficLightRoadSideNL_4_Casing.LightGreen_Power  Value=0
  TrafficLightRoadSideNL_4_Casing.LightGreen_SPDIndex : Constant  Tag=TrafficLightRoadSideNL_4_Casing.LightGreen_SPDIndex  Value=15
  TrafficLightRoadSideNL_4_Casing.LightOrange_Control_Mux : Subsystem  Tag=mux/plugin/LightSignals
  TrafficLightRoadSideNL_4_Casing.LightOrange_Power : Constant  Tag=TrafficLightRoadSideNL_4_Casing.LightOrange_Power  Value=0
  TrafficLightRoadSideNL_4_Casing.LightOrange_SPDIndex : Constant  Tag=TrafficLightRoadSideNL_4_Casing.LightOrange_SPDIndex  Value=14
  TrafficLightRoadSideNL_4_Casing.LightRed_Control_Mux : Subsystem  Tag=mux/plugin/LightSignals
  TrafficLightRoadSideNL_4_Casing.LightRed_Power : Constant  Tag=TrafficLightRoadSideNL_4_Casing.LightRed_Power  Value=0
  TrafficLightRoadSideNL_4_Casing.LightRed_SPDIndex : Constant  Tag=TrafficLightRoadSideNL_4_Casing.LightRed_SPDIndex  Value=16
  VISUCasingLights_Mux : Subsystem  Tag=mux/VisuCasingLights  mask(PreScan User Interface: VisuTrafficLight){}
      mask help:
      | The VisuTrafficLight block provides a way to animate traffic lights: switch on and off individual lights.
      |
      | For more information, please click Help.
      mask Help: eval('openHelp(731)')
  VISUCasingLights_TrafficLightRoadSideNL_4 : Outport  Tag=outport/VisuCasingLights  SampleTime=1/300
  TrafficLightRoadSideNL_4_Casing.LightRed_Control : Outport  Tag=outport/plugin/sfun_PBCLight  Port=2  OutDataTypeStr=Bus: PRESCAN_PBCLIGHT_DATA  PortDimensions=1  SampleTime=0.05
  TrafficLightRoadSideNL_4_Casing.LightOrange_Control : Outport  Tag=outport/plugin/sfun_PBCLight  Port=3  OutDataTypeStr=Bus: PRESCAN_PBCLIGHT_DATA  PortDimensions=1  SampleTime=0.05
  TrafficLightRoadSideNL_4_Casing.LightGreen_Control : Outport  Tag=outport/plugin/sfun_PBCLight  Port=4  OutDataTypeStr=Bus: PRESCAN_PBCLIGHT_DATA  PortDimensions=1  SampleTime=0.05
  wires:
  VISUCasingLights_Mux/1(VISUCasingLights_TrafficLightRoadSideNL_4) -> VISUCasingLights_TrafficLightRoadSideNL_4/1
  TrafficLightRoadSideNL_4_Casing.LightRed_Control_Mux/1(Bus) -> TrafficLightRoadSideNL_4_Casing.LightRed_Control/1
  TrafficLightRoadSideNL_4_Casing.LightRed_SPDIndex/1 -> TrafficLightRoadSideNL_4_Casing.LightRed_Control_Mux/1(SPDIndex [-])
  TrafficLightRoadSideNL_4_Casing.LightRed_Power/1 -> TrafficLightRoadSideNL_4_Casing.LightRed_Control_Mux/2(Power [W])
  TrafficLightRoadSideNL_4_Casing.LightOrange_Control_Mux/1(Bus) -> TrafficLightRoadSideNL_4_Casing.LightOrange_Control/1
  TrafficLightRoadSideNL_4_Casing.LightOrange_SPDIndex/1 -> TrafficLightRoadSideNL_4_Casing.LightOrange_Control_Mux/1(SPDIndex [-])
  TrafficLightRoadSideNL_4_Casing.LightOrange_Power/1 -> TrafficLightRoadSideNL_4_Casing.LightOrange_Control_Mux/2(Power [W])
  TrafficLightRoadSideNL_4_Casing.LightGreen_Control_Mux/1(Bus) -> TrafficLightRoadSideNL_4_Casing.LightGreen_Control/1
  TrafficLightRoadSideNL_4_Casing.LightGreen_SPDIndex/1 -> TrafficLightRoadSideNL_4_Casing.LightGreen_Control_Mux/1(SPDIndex [-])
  TrafficLightRoadSideNL_4_Casing.LightGreen_Power/1 -> TrafficLightRoadSideNL_4_Casing.LightGreen_Control_Mux/2(Power [W])
  Ground_1/1 -> VISUCasingLights_Mux/1(Green [-])
  Ground_2/1 -> VISUCasingLights_Mux/2(Orange [-])
  Ground_3/1 -> VISUCasingLights_Mux/3(Red [-])

== system Base_Map_cs/TrafficLightRoadSideNL_4_Casing.LightGreen_Control ==
  TrafficLightRoadSideNL_4_Casing.LightGreen_Control : Inport  Tag=inport/plugin/sfun_PBCLight  OutDataTypeStr=Bus: PRESCAN_PBCLIGHT_DATA  PortDimensions=1  SampleTime=0.05  BusOutputAsStruct=on
  Actuator : S-Function  LoadFcn=addpath 'C:/Program Files/Simcenter Prescan/Prescan_2019.1/Plugins/PBCameraPlugin/matlab';addpath 'C:/Program Files/Simcenter Prescan/Prescan_2019.1/Plugins/PBCameraPlugin/bin';load('PreScanPBCLightData.mat');  FunctionName=sfun_PBCLight  Parameters=lightID, timestepMask  SFunctionDeploymentMode=off  EnableBusSupport=off  mask(Physics Based Camera plugin block){lightID=11, timestepMask=0.05}
      mask prompts: lightID "Light ID:"; timestepMask "MATLAB timestep:"
      mask help: Light Control I/O
      mask Help: eval('openHelp(6500)')
      mask Display: image(imread('ico_PBCControl.png'))
  wires:
  TrafficLightRoadSideNL_4_Casing.LightGreen_Control/1 -> Actuator/1

== system Base_Map_cs/TrafficLightRoadSideNL_4_Casing.LightOrange_Control ==
  TrafficLightRoadSideNL_4_Casing.LightOrange_Control : Inport  Tag=inport/plugin/sfun_PBCLight  OutDataTypeStr=Bus: PRESCAN_PBCLIGHT_DATA  PortDimensions=1  SampleTime=0.05  BusOutputAsStruct=on
  Actuator : S-Function  LoadFcn=addpath 'C:/Program Files/Simcenter Prescan/Prescan_2019.1/Plugins/PBCameraPlugin/matlab';addpath 'C:/Program Files/Simcenter Prescan/Prescan_2019.1/Plugins/PBCameraPlugin/bin';load('PreScanPBCLightData.mat');  FunctionName=sfun_PBCLight  Parameters=lightID, timestepMask  SFunctionDeploymentMode=off  EnableBusSupport=off  mask(Physics Based Camera plugin block){lightID=10, timestepMask=0.05}
      mask prompts: lightID "Light ID:"; timestepMask "MATLAB timestep:"
      mask help: Light Control I/O
      mask Help: eval('openHelp(6500)')
      mask Display: image(imread('ico_PBCControl.png'))
  wires:
  TrafficLightRoadSideNL_4_Casing.LightOrange_Control/1 -> Actuator/1

== system Base_Map_cs/TrafficLightRoadSideNL_4_Casing.LightRed_Control ==
  TrafficLightRoadSideNL_4_Casing.LightRed_Control : Inport  Tag=inport/plugin/sfun_PBCLight  OutDataTypeStr=Bus: PRESCAN_PBCLIGHT_DATA  PortDimensions=1  SampleTime=0.05  BusOutputAsStruct=on
  Actuator : S-Function  LoadFcn=addpath 'C:/Program Files/Simcenter Prescan/Prescan_2019.1/Plugins/PBCameraPlugin/matlab';addpath 'C:/Program Files/Simcenter Prescan/Prescan_2019.1/Plugins/PBCameraPlugin/bin';load('PreScanPBCLightData.mat');  FunctionName=sfun_PBCLight  Parameters=lightID, timestepMask  SFunctionDeploymentMode=off  EnableBusSupport=off  mask(Physics Based Camera plugin block){lightID=9, timestepMask=0.05}
      mask prompts: lightID "Light ID:"; timestepMask "MATLAB timestep:"
      mask help: Light Control I/O
      mask Help: eval('openHelp(6500)')
      mask Display: image(imread('ico_PBCControl.png'))
  wires:
  TrafficLightRoadSideNL_4_Casing.LightRed_Control/1 -> Actuator/1

== system Base_Map_cs/TrafficLightRoadSideNL_5 ==
  note: Light SPD Resources
      |
      |  0: CIE_A_standard_incandescent_illuminant.txt
      |  1: CIE_A_standard_incandescent_illuminant.txt_x_R255_G191_B000.txt
      |  2: CIE_A_standard_incandescent_illuminant.txt_x_R583_G047_B000.txt
      |  3: CIE_F12_standard_fluorescent_illuminant.txt
      |  4: Illuminant_D65.txt
      |  5: Light_SPD_H1_12_8V_Filament.txt
      |  6: Light_SPD_H1_13_2V_Filament.txt
      |  7: Light_SPD_H11_12V_Filament.txt
      |  8: Light_SPD_H7_12_8V_Filament.txt
      |  9: Light_SPD_H7_13_2V_Filament.txt
      | 10: Light_SPD_H8_13_2V_Filament.txt
      | 11: Light_SPD_Halogen.txt
      | 12: Light_SPD_High_Power_LED.txt
      | 13: Light_SPD_HPS_High_Pressure_Sodium.txt
      | 14: Light_SPD_incandescent_traffic_signal_amber.txt
      | 15: Light_SPD_incandescent_traffic_signal_green.txt
      | 16: Light_SPD_incandescent_traffic_signal_red.txt
      | 17: Light_SPD_LED_D1S_HID.txt
      | 18: Light_SPD_LED_traffic_signal_amber.txt
      | 19: Light_SPD_LED_traffic_signal_green.txt
      | 20: Light_SPD_LED_traffic_signal_red.txt
      | 21: Light_SPD_LPS_Low_Pressure_Sodium.txt
      | 22: Light_SPD_Mercury.txt
      | 23: Light_SPD_Reddish_Neon_Sign.txt
      | 24: Noma_Twister_Blue_13W_120V.txt
      | 25: Philips_Blue_Golite_P1_Apollo_1750Lux.txt
      | 26: SPD_flat_1.0.txt
  note: Light SPD Resources
  Ground_1 : Ground
  Ground_2 : Ground
  Ground_3 : Ground
  TrafficLightRoadSideNL_5_Casing.LightGreen_Control_Mux : Subsystem  Tag=mux/plugin/LightSignals
  TrafficLightRoadSideNL_5_Casing.LightGreen_Power : Constant  Tag=TrafficLightRoadSideNL_5_Casing.LightGreen_Power  Value=0
  TrafficLightRoadSideNL_5_Casing.LightGreen_SPDIndex : Constant  Tag=TrafficLightRoadSideNL_5_Casing.LightGreen_SPDIndex  Value=15
  TrafficLightRoadSideNL_5_Casing.LightOrange_Control_Mux : Subsystem  Tag=mux/plugin/LightSignals
  TrafficLightRoadSideNL_5_Casing.LightOrange_Power : Constant  Tag=TrafficLightRoadSideNL_5_Casing.LightOrange_Power  Value=0
  TrafficLightRoadSideNL_5_Casing.LightOrange_SPDIndex : Constant  Tag=TrafficLightRoadSideNL_5_Casing.LightOrange_SPDIndex  Value=14
  TrafficLightRoadSideNL_5_Casing.LightRed_Control_Mux : Subsystem  Tag=mux/plugin/LightSignals
  TrafficLightRoadSideNL_5_Casing.LightRed_Power : Constant  Tag=TrafficLightRoadSideNL_5_Casing.LightRed_Power  Value=0
  TrafficLightRoadSideNL_5_Casing.LightRed_SPDIndex : Constant  Tag=TrafficLightRoadSideNL_5_Casing.LightRed_SPDIndex  Value=16
  VISUCasingLights_Mux : Subsystem  Tag=mux/VisuCasingLights  mask(PreScan User Interface: VisuTrafficLight){}
      mask help:
      | The VisuTrafficLight block provides a way to animate traffic lights: switch on and off individual lights.
      |
      | For more information, please click Help.
      mask Help: eval('openHelp(731)')
  VISUCasingLights_TrafficLightRoadSideNL_5 : Outport  Tag=outport/VisuCasingLights  SampleTime=1/300
  TrafficLightRoadSideNL_5_Casing.LightRed_Control : Outport  Tag=outport/plugin/sfun_PBCLight  Port=2  OutDataTypeStr=Bus: PRESCAN_PBCLIGHT_DATA  PortDimensions=1  SampleTime=0.05
  TrafficLightRoadSideNL_5_Casing.LightOrange_Control : Outport  Tag=outport/plugin/sfun_PBCLight  Port=3  OutDataTypeStr=Bus: PRESCAN_PBCLIGHT_DATA  PortDimensions=1  SampleTime=0.05
  TrafficLightRoadSideNL_5_Casing.LightGreen_Control : Outport  Tag=outport/plugin/sfun_PBCLight  Port=4  OutDataTypeStr=Bus: PRESCAN_PBCLIGHT_DATA  PortDimensions=1  SampleTime=0.05
  wires:
  VISUCasingLights_Mux/1(VISUCasingLights_TrafficLightRoadSideNL_5) -> VISUCasingLights_TrafficLightRoadSideNL_5/1
  TrafficLightRoadSideNL_5_Casing.LightRed_Control_Mux/1(Bus) -> TrafficLightRoadSideNL_5_Casing.LightRed_Control/1
  TrafficLightRoadSideNL_5_Casing.LightRed_SPDIndex/1 -> TrafficLightRoadSideNL_5_Casing.LightRed_Control_Mux/1(SPDIndex [-])
  TrafficLightRoadSideNL_5_Casing.LightRed_Power/1 -> TrafficLightRoadSideNL_5_Casing.LightRed_Control_Mux/2(Power [W])
  TrafficLightRoadSideNL_5_Casing.LightOrange_Control_Mux/1(Bus) -> TrafficLightRoadSideNL_5_Casing.LightOrange_Control/1
  TrafficLightRoadSideNL_5_Casing.LightOrange_SPDIndex/1 -> TrafficLightRoadSideNL_5_Casing.LightOrange_Control_Mux/1(SPDIndex [-])
  TrafficLightRoadSideNL_5_Casing.LightOrange_Power/1 -> TrafficLightRoadSideNL_5_Casing.LightOrange_Control_Mux/2(Power [W])
  TrafficLightRoadSideNL_5_Casing.LightGreen_Control_Mux/1(Bus) -> TrafficLightRoadSideNL_5_Casing.LightGreen_Control/1
  TrafficLightRoadSideNL_5_Casing.LightGreen_SPDIndex/1 -> TrafficLightRoadSideNL_5_Casing.LightGreen_Control_Mux/1(SPDIndex [-])
  TrafficLightRoadSideNL_5_Casing.LightGreen_Power/1 -> TrafficLightRoadSideNL_5_Casing.LightGreen_Control_Mux/2(Power [W])
  Ground_1/1 -> VISUCasingLights_Mux/1(Green [-])
  Ground_2/1 -> VISUCasingLights_Mux/2(Orange [-])
  Ground_3/1 -> VISUCasingLights_Mux/3(Red [-])

== system Base_Map_cs/TrafficLightRoadSideNL_5_Casing.LightGreen_Control ==
  TrafficLightRoadSideNL_5_Casing.LightGreen_Control : Inport  Tag=inport/plugin/sfun_PBCLight  OutDataTypeStr=Bus: PRESCAN_PBCLIGHT_DATA  PortDimensions=1  SampleTime=0.05  BusOutputAsStruct=on
  Actuator : S-Function  LoadFcn=addpath 'C:/Program Files/Simcenter Prescan/Prescan_2019.1/Plugins/PBCameraPlugin/matlab';addpath 'C:/Program Files/Simcenter Prescan/Prescan_2019.1/Plugins/PBCameraPlugin/bin';load('PreScanPBCLightData.mat');  FunctionName=sfun_PBCLight  Parameters=lightID, timestepMask  SFunctionDeploymentMode=off  EnableBusSupport=off  mask(Physics Based Camera plugin block){lightID=14, timestepMask=0.05}
      mask prompts: lightID "Light ID:"; timestepMask "MATLAB timestep:"
      mask help: Light Control I/O
      mask Help: eval('openHelp(6500)')
      mask Display: image(imread('ico_PBCControl.png'))
  wires:
  TrafficLightRoadSideNL_5_Casing.LightGreen_Control/1 -> Actuator/1
